simulink model "DoubleMotorExperiment"  (R2020a)
settings: Solver=FixedStepAuto  StartTime=0.0  StopTime=10.0  RelTol=1e-3
InitFcn:
  | %Motor1 = Epos4(1,0);
  | %Motor2 = Epos4(2,0);
model workspace (MAT data in the model file):
  NodeID = 1
  OperationMode = 0
  Ts = 0.001
CloseFcn:
  | %delete(Motor1);
  | %delete(Motor2);
settings Model: DataDictionary=MotorInfo.sldd  Creator=khoi  LastModifiedBy=khoi
settings RTWCC: GenCodeOnly=on

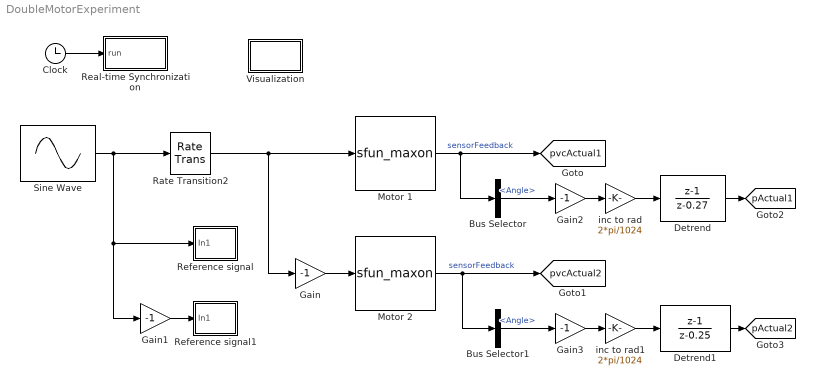
== system DoubleMotorExperiment ==
  Bus Selector : BusSelector  OutputSignals=Angle
  Bus Selector1 : BusSelector  OutputSignals=Angle
  Clock : Clock
  Detrend : DiscreteTransferFcn  Numerator=[1 -1]  Denominator=[1 -0.27]
  Detrend1 : DiscreteTransferFcn  Numerator=[1 -1]  Denominator=[1 -0.25]
  Gain{,1..3} (4 alike) : Gain  Gain=-1
  Motor 1 : S-Function  FunctionName=sfun_maxon  Parameters=NodeID, DeltaT, OpMode  SFunctionDeploymentMode=off  EnableBusSupport=off  mask{NodeID=1, DeltaT=0.02, OpMode=Cyclic synchronous velocity mode, P_cur=0, I_cur=0, P_pos=0, I_pos=0, D_pos=0, v_posGainFF=0, a_posGainFF=0, P_vel=0, I_vel=0, v_velGainFF=0, a_velGainFF=0, f_velCutoff=0}
      mask prompts: NodeID "Node ID"; DeltaT "Sample time (s)"; OpMode "Operation mode"; P_cur "P gain"; I_cur "I gain"; P_pos "P gain"; I_pos "I gain"; D_pos "D gain"; v_posGainFF "FF velocity gain"; a_posGainFF "FF acceleration gain"; P_vel "P gain"; I_vel "I gain"; v_velGainFF "Feed-forward velocity gain"; a_velGainFF "Feed-forward acceleration gain"; f_velCutoff "Filter cut-off frequency"
      mask TypeOptions OpMode: Cyclic synchronous current (torque) mode | Cyclic synchronous velocity mode | Cyclic synchronous position mode | Profile velocity mode | Profile position mode
      mask DialogControl DescGroupVar Prompt: Motor Parameters
      mask DialogControl DescTextVar Prompt: The block outputs MotorInfo bus signal, which consists of the following variables: angle (increment), speed (rpm), current (mA)
      mask DialogControl Container6 Prompt: Motor
      mask DialogControl Container14 Prompt: Controller Parameters
      mask DialogControl DescTextVar_copy Prompt: This tab is experimental and does not implemented yet. Changing these parameters will not affect the motor performance.
      mask DialogControl Container15 Prompt: Current controller parameter set
      mask DialogControl Container15_copy Prompt: Position controller parameter set
      mask DialogControl Container15_copy_copy Prompt: Velocity controller parameter set
      mask Display:
      | disp('Maxon motor\nHIL');
      | % port_label('input', 1, 'inputSignal');
      | % port_label('output', 1, 'SENSR');
  Motor 2 : S-Function  FunctionName=sfun_maxon  Parameters=NodeID, DeltaT, OpMode  SFunctionDeploymentMode=off  EnableBusSupport=off  mask{NodeID=2, DeltaT=0.02, OpMode=Cyclic synchronous velocity mode, P_cur=0, I_cur=0, P_pos=0, I_pos=0, D_pos=0, v_posGainFF=0, a_posGainFF=0, P_vel=0, I_vel=0, v_velGainFF=0, a_velGainFF=0, f_velCutoff=0}
      mask prompts: NodeID "Node ID"; DeltaT "Sample time"; OpMode "Operation mode"; P_cur "P gain"; I_cur "I gain"; P_pos "P gain"; I_pos "I gain"; D_pos "D gain"; v_posGainFF "FF velocity gain"; a_posGainFF "FF acceleration gain"; P_vel "P gain"; I_vel "I gain"; v_velGainFF "Feed-forward velocity gain"; a_velGainFF "Feed-forward acceleration gain"; f_velCutoff "Filter cut-off frequency"
      mask TypeOptions OpMode: Cyclic synchronous current (torque) mode | Cyclic synchronous velocity mode | Cyclic synchronous position mode | Profile velocity mode | Profile position mode
      mask DialogControl DescGroupVar Prompt: Motor Parameters
      mask DialogControl Container6 Prompt: Motor
      mask DialogControl Container14 Prompt: Controller Parameters
      mask DialogControl DescTextVar_copy Prompt: This tab is experimental and does not implemented yet. Changing these parameters will not affect the motor performance.
      mask DialogControl Container15 Prompt: Current controller parameter set
      mask DialogControl Container15_copy Prompt: Position controller parameter set
      mask DialogControl Container15_copy_copy Prompt: Velocity controller parameter set
      mask Display:
      | disp('Maxon motor\nHIL');
      | % port_label('input', 1, 'inputSignal');
      | % port_label('output', 1, 'SENSR');
  Rate Transition2 : RateTransition  OutPortSampleTime=0.1
  Real-time Synchronization : Subsystem
  Reference signal : Subsystem
  Reference signal1 : Subsystem
  Sine Wave : Sin  Amplitude=2000  Frequency=10  SampleTime=0
  Visualization : Subsystem
  inc to rad : Gain  Gain=2*pi/1024
  inc to rad1 : Gain  Gain=2*pi/1024
  tag scope: pActual1=global, pActual2=global, pvcActual1=global, pvcActual2=global
  wires:
  Clock/1 -> Real-time Synchronization/1(run)
  Motor 2/1 -> [pvcActual2], Bus Selector1/1  "sensorFeedback"
  Rate Transition2/1 -> Motor 1/1, Gain/1
  Gain/1 -> Motor 2/1
  Motor 1/1 -> [pvcActual1], Bus Selector/1  "sensorFeedback"
  Bus Selector/1 -> Gain2/1  "<Angle>"
  inc to rad/1 -> Detrend/1
  inc to rad1/1 -> Detrend1/1
  Bus Selector1/1 -> Gain3/1  "<Angle>"
  Sine Wave/1 -> Gain1/1, Reference signal/1(In1), Rate Transition2/1
  Gain2/1 -> inc to rad/1
  Gain3/1 -> inc to rad1/1
  Gain1/1 -> Reference signal1/1(In1)
  Detrend1/1 -> [pActual2]
  Detrend/1 -> [pActual1]

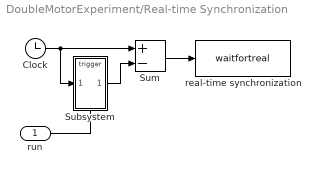
== system DoubleMotorExperiment/Real-time Synchronization ==
  run : Inport
  Clock : Clock
  Subsystem : Subsystem  TreatAsAtomicUnit=on
  Sum : Sum  Inputs=+-  InputSameDT=on  SaturateOnIntegerOverflow=on  OutDataTypeStr=Inherit: Same as first input
  real-time synchronization : MATLABFcn  MATLABFcn=waitfortreal  OutputDimensions=0
  wires:
  Clock/1 -> Subsystem/1(In), Sum/1
  Subsystem/1(Out) -> Sum/2
  Sum/1 -> real-time synchronization/1
  run/1 -> Subsystem/Trigger

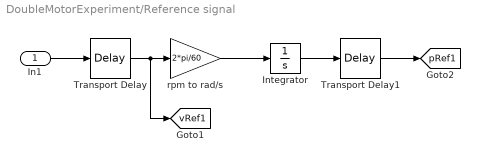
== system DoubleMotorExperiment/Reference signal ==
  In1 : Inport
  Integrator : Integrator  InitialCondition=-2000*2*pi/60*0.1
  Transport Delay : TransportDelay  DelayTime=0.1
  Transport Delay1 : TransportDelay  DelayTime=0.2
  rpm to rad/s : Gain  Gain=2*pi/60
  tag scope: pRef1=global, vRef1=global
  wires:
  Transport Delay/1 -> [vRef1], rpm to rad/s/1
  rpm to rad/s/1 -> Integrator/1
  Integrator/1 -> Transport Delay1/1
  Transport Delay1/1 -> [pRef1]
  In1/1 -> Transport Delay/1

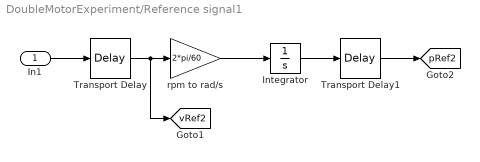
== system DoubleMotorExperiment/Reference signal1 ==
  In1 : Inport
  Integrator : Integrator  InitialCondition=2000*2*pi/60*0.1
  Transport Delay : TransportDelay  DelayTime=0.1
  Transport Delay1 : TransportDelay  DelayTime=0.2
  rpm to rad/s : Gain  Gain=2*pi/60
  tag scope: pRef2=global, vRef2=global
  wires:
  In1/1 -> Transport Delay/1
  Transport Delay1/1 -> [pRef2]
  Integrator/1 -> Transport Delay1/1
  rpm to rad/s/1 -> Integrator/1
  Transport Delay/1 -> rpm to rad/s/1, [vRef2]

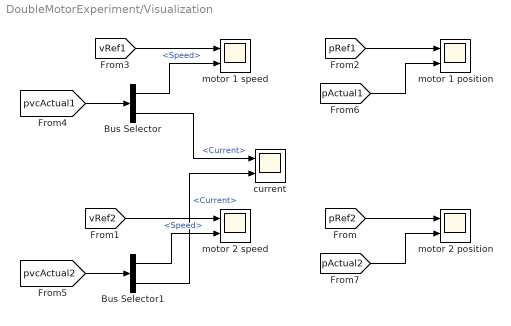
== system DoubleMotorExperiment/Visualization ==
  Bus Selector : BusSelector  OutputSignals=Speed,Current
  Bus Selector1 : BusSelector  OutputSignals=Speed,Current
  current : Scope  NumInputPorts=2
  motor 1 position : Scope  NumInputPorts=2
  motor 1 speed : Scope  NumInputPorts=2
  motor 2 position : Scope  NumInputPorts=2
  motor 2 speed : Scope  NumInputPorts=2
  wires:
  [pActual1] -> motor 1 position/2
  [vRef2] -> motor 2 speed/1
  [pvcActual2] -> Bus Selector1/1
  [pRef2] -> motor 2 position/1
  [pvcActual1] -> Bus Selector/1
  [pRef1] -> motor 1 position/1
  [vRef1] -> motor 1 speed/1
  [pActual2] -> motor 2 position/2
  Bus Selector1/1 -> motor 2 speed/2  "<Speed>"
  Bus Selector/1 -> motor 1 speed/2  "<Speed>"
  Bus Selector/2 -> current/1  "<Current>"
  Bus Selector1/2 -> current/2  "<Current>"

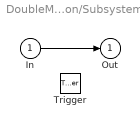
== system DoubleMotorExperiment/Real-time Synchronization/Subsystem ==
  In : Inport
  Trigger : TriggerPort  VariantControl=(inherit)
  Out : Outport  InitialOutput=0
  wires:
  In/1 -> Out/1
